simulink model "Car_Blinkers_2020b"  (R2020b)
settings: Solver=FixedStepDiscrete  StartTime=0.0  StopTime=10.0  FixedStep=1e-3  RelTol=1e-3
libraries: arduinolib x5, dspswit3 x3
settings Model: SILPILModeSetting=veronly  ExtModeTrigDuration=2  Creator=gaafa  LastModifiedBy=gaafa
settings SolverCC: AutoInsertRateTranBlk=on
settings OptimizationCC: UseDivisionForNetSlopeComputation=on  GainParamInheritBuiltInType=on  UseFloatMulNetSlope=on  PassReuseOutputArgsAs=Individual arguments  ZeroExternalMemoryAtStartup=off  ZeroInternalMemoryAtStartup=off  NoFixptDivByZeroProtection=on  EfficientFloat2IntCast=on  LifeSpan=1  MaxStackSize=64  OptimizeBlockOrder=speed  DifferentSizesBufferReuse=on  EfficientTunableParamExpr=on
settings DebuggingCC: ParameterTunabilityLossMsg=error  UnconnectedInputMsg=none  UnconnectedOutputMsg=none  UnconnectedLineMsg=none
settings HardwareCC: ProdBitPerInt=16  ProdBitPerPointer=16  ProdBitPerSizeT=16  ProdBitPerPtrDiffT=16  ProdLargestAtomicFloat=None  ProdWordSize=8  ProdHWDeviceType=Atmel->AVR
settings ModelReferenceCC: EnableRefExpFcnMdlSchedulingChecks=off
settings SFSimCC: MATLABDynamicMemAlloc=off
settings RTWCC: Description=Embedded Coder  SystemTargetFile=ert.tlc  HardwareBoard=Arduino Uno  TemplateMakefile=ert_default_tmf  Toolchain=Arduino AVR  BuildConfiguration=Faster Runs
settings CodeAppCC: ForceParamTrailComments=on  IgnoreCustomStorageClasses=off  OperatorAnnotations=on  SimulinkDataObjDesc=on  SFDataObjDesc=on  CustomSymbolStrGlobalVar=rt$N$M  CustomSymbolStrType=$N$M  CustomSymbolStrFcn=$N$M$F  CustomSymbolStrMacro=$N$M  InsertBlockDesc=on
settings ERTTargetCC: IncludeMdlTerminateFcn=off  CombineSignalStateStructs=on  SupportAbsoluteTime=off  SupportComplex=off  SupportContinuousTime=on  SupportNonInlinedSFcns=on  SupportVariableSizeSignals=on  ExtModeTransport=3  ExtModeStaticAlloc=on  ExtModeStaticAllocSize=250  ExtModeMexFile=ext_xcp  ExtModeIntrfLevel=Level2 - Open  ERTFilePackagingFormat=CompactWithDataFile

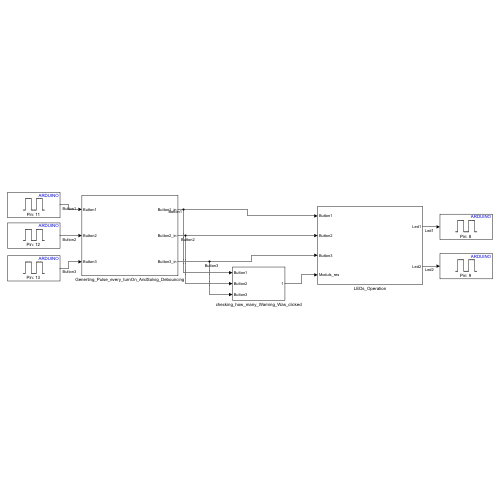
[thumbnail: Simulink's stored preview of the top-level diagram]
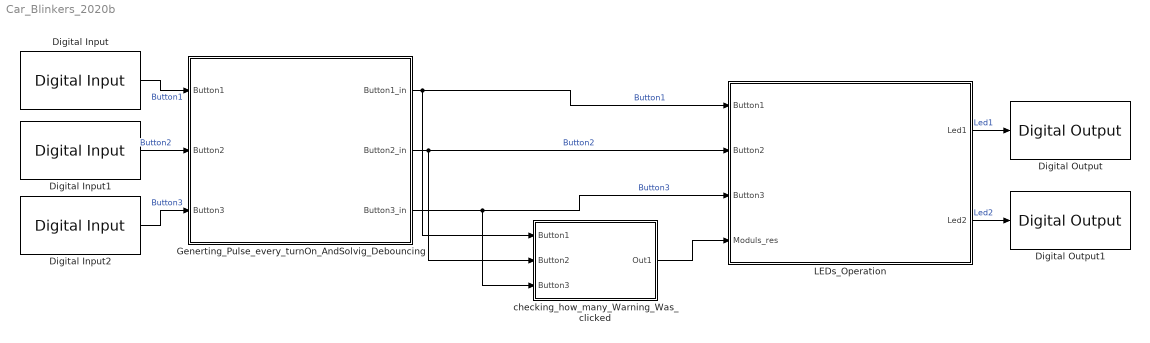
== system Car_Blinkers_2020b ==
  Digital Input : arduinolib/Digital Input  pinNumber=11  mode=Default  Direction=input  SampleTime=0.1  blockPlatform=arduino
  Digital Input1 : arduinolib/Digital Input  pinNumber=12  mode=Default  Direction=input  SampleTime=0.1  blockPlatform=arduino
  Digital Input2 : arduinolib/Digital Input  pinNumber=13  mode=Default  Direction=input  SampleTime=0.1  blockPlatform=arduino
  Digital Output : arduinolib/Digital Output  pinNumber=8  Direction=output  blockPlatform=arduino
  Digital Output1 : arduinolib/Digital Output  pinNumber=9  Direction=output  blockPlatform=arduino
  Generting_Pulse_every_turnOn_AndSolvig_Debouncing : Subsystem
  LEDs_Operation : Subsystem
  checking_how_many_Warning_Was_clicked : Subsystem
  wires:
  Digital Input/1 -> Generting_Pulse_every_turnOn_AndSolvig_Debouncing/1(Button1)  "Button1"
  Digital Input1/1 -> Generting_Pulse_every_turnOn_AndSolvig_Debouncing/2(Button2)  "Button2"
  LEDs_Operation/1(Led1) -> Digital Output/1  "Led1"
  Generting_Pulse_every_turnOn_AndSolvig_Debouncing/3(Button3_in) -> LEDs_Operation/3(Button3), checking_how_many_Warning_Was_clicked/3(Button3)  "Button3"
  Generting_Pulse_every_turnOn_AndSolvig_Debouncing/2(Button2_in) -> LEDs_Operation/2(Button2), checking_how_many_Warning_Was_clicked/2(Button2)  "Button2"
  Digital Input2/1 -> Generting_Pulse_every_turnOn_AndSolvig_Debouncing/3(Button3)  "Button3"
  Generting_Pulse_every_turnOn_AndSolvig_Debouncing/1(Button1_in) -> checking_how_many_Warning_Was_clicked/1(Button1), LEDs_Operation/1(Button1)  "Button1"
  checking_how_many_Warning_Was_clicked/1(Out1) -> LEDs_Operation/4(Moduls_res)
  LEDs_Operation/2(Led2) -> Digital Output1/1  "Led2"

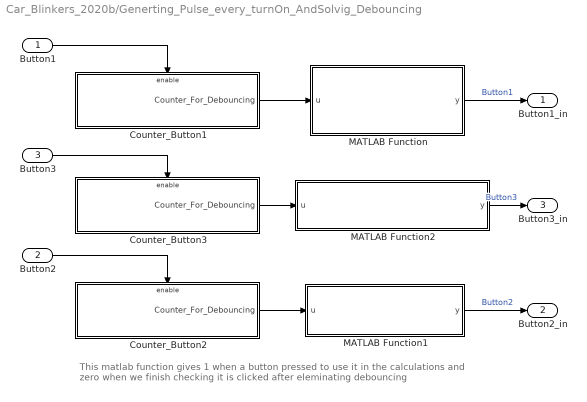
== system Car_Blinkers_2020b/Generting_Pulse_every_turnOn_AndSolvig_Debouncing ==
  note: This matlab function gives 1 when a button pressed to use it in the calculations
      | and zero when we finish checking it is clicked after eleminating debouncing
  Button1 : Inport
  Button2 : Inport  Port=2
  Button3 : Inport  Port=3
  Counter_Button1 : Subsystem  TreatAsAtomicUnit=on
  Counter_Button2 : Subsystem  TreatAsAtomicUnit=on
  Counter_Button3 : Subsystem  TreatAsAtomicUnit=on
  MATLAB Function : MATLAB Function  TreatAsAtomicUnit=on
  MATLAB Function1 : MATLAB Function  TreatAsAtomicUnit=on
  MATLAB Function2 : MATLAB Function  TreatAsAtomicUnit=on
  Button1_in : Outport
  Button2_in : Outport  Port=2
  Button3_in : Outport  Port=3
  wires:
  Counter_Button1/1(Counter_For_Debouncing) -> MATLAB Function/1(u)
  Button2/1 -> Counter_Button2/Enable
  Button3/1 -> Counter_Button3/Enable
  Button1/1 -> Counter_Button1/Enable
  Counter_Button3/1(Counter_For_Debouncing) -> MATLAB Function2/1(u)
  MATLAB Function2/1(y) -> Button3_in/1  "Button3"
  MATLAB Function/1(y) -> Button1_in/1  "Button1"
  Counter_Button2/1(Counter_For_Debouncing) -> MATLAB Function1/1(u)
  MATLAB Function1/1(y) -> Button2_in/1  "Button2"

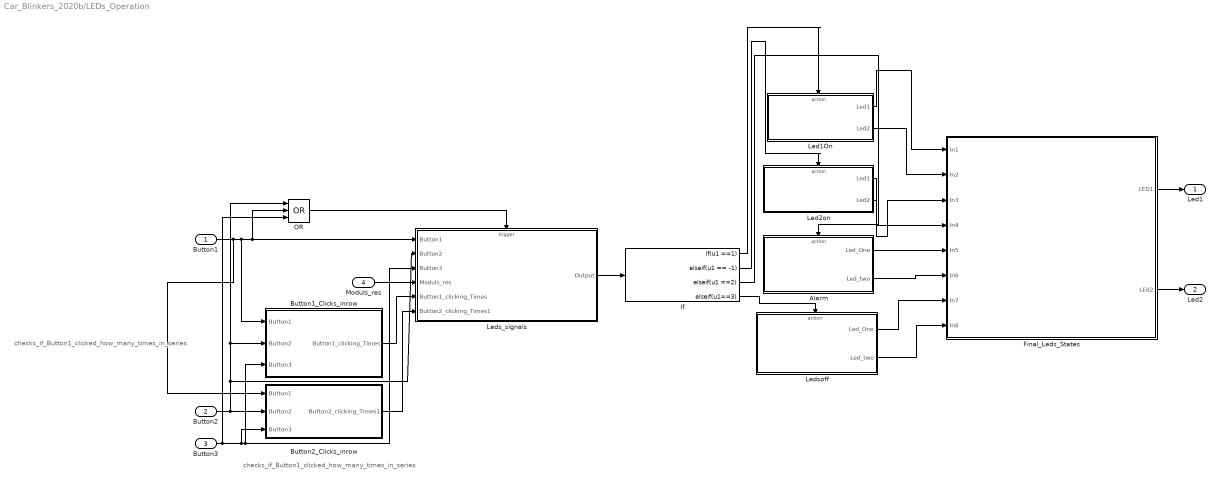
== system Car_Blinkers_2020b/LEDs_Operation ==
  note: checks_if_Button1_clicked_how_many_times_in_series
  note: checks_if_Button1_clicked_how_many_times_in_series
  Button1 : Inport
  Button2 : Inport  Port=2
  Button3 : Inport  Port=3
  Moduls_res : Inport  Port=4
  Alarm : Subsystem  TreatAsAtomicUnit=on
  Button1_Clicks_inrow : Subsystem
  Button2_Clicks_inrow : Subsystem
  Final_Leds_States : Subsystem
  If : If  IfExpression=u1 ==1  ElseIfExpressions=u1 == -1 , u1 ==2 , u1==3  ShowElse=off
  Led1On : Subsystem  TreatAsAtomicUnit=on
  Led2on : Subsystem  TreatAsAtomicUnit=on
  Leds_signals : Subsystem  TreatAsAtomicUnit=on
  Ledsoff : Subsystem  TreatAsAtomicUnit=on
  OR : Logic  Operator=OR  Inputs=3  IconShape=distinctive  AllPortsSameDT=off  OutDataTypeStr=boolean
  Led1 : Outport
  Led2 : Outport  Port=2
  wires:
  If/4 -> Ledsoff/Action
  Button1/1 -> OR/2, Leds_signals/1(Button1), Button1_Clicks_inrow/1(Button1), Button2_Clicks_inrow/1(Button1)
  Moduls_res/1 -> Leds_signals/4(Moduls_res)
  Button2/1 -> Button1_Clicks_inrow/2(Button2), OR/1, Leds_signals/2(Button2), Button2_Clicks_inrow/2(Button2)
  Leds_signals/1(Output) -> If/1
  Button2_Clicks_inrow/1(Button2_clicking_Times1) -> Leds_signals/6(Button2_clicking_Times1)
  Button3/1 -> Button1_Clicks_inrow/3(Button3), Leds_signals/3(Button3), Button2_Clicks_inrow/3(Button3), OR/3
  OR/1 -> Leds_signals/Trigger
  Final_Leds_States/1(LED1) -> Led1/1
  Led2on/2(Led2) -> Final_Leds_States/4(In4)
  Button1_Clicks_inrow/1(Button1_clicking_Times) -> Leds_signals/5(Button1_clicking_Times)
  If/1 -> Led1On/Action
  Alarm/2(Led_two) -> Final_Leds_States/6(In6)
  If/2 -> Led2on/Action
  If/3 -> Alarm/Action
  Ledsoff/2(Led_two) -> Final_Leds_States/8(In8)
  Led1On/1(Led1) -> Final_Leds_States/1(In1)
  Led1On/2(Led2) -> Final_Leds_States/2(In2)
  Led2on/1(Led1) -> Final_Leds_States/3(In3)
  Alarm/1(Led_One) -> Final_Leds_States/5(In5)
  Ledsoff/1(Led_One) -> Final_Leds_States/7(In7)
  Final_Leds_States/2(LEd2) -> Led2/1

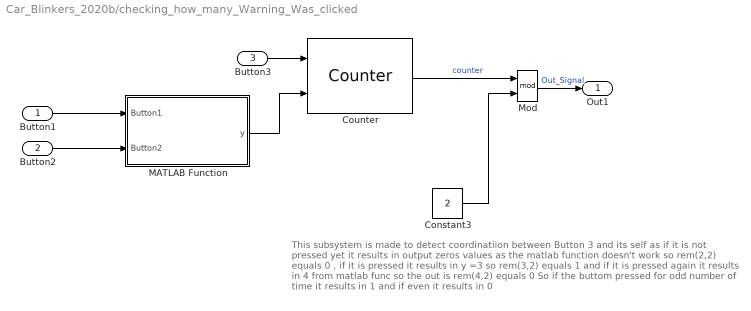
== system Car_Blinkers_2020b/checking_how_many_Warning_Was_clicked ==
  note: This subsystem is made to detect coordinatiion between Button 3 and its self as if it is not pressed yet it results in output zeros values as the matlab function doesn't work
      | so rem(2,2) equals 0 , if it is pressed it results in y =3 so rem(3,2) equals 1 and if it is pressed again it results in 4 from matlab func so the out is rem(4,2) equals 0
      | So if the buttom pressed for odd number of time it results in 1 and if even it results in 0
  Button1 : Inport
  Button2 : Inport  Port=2
  Button3 : Inport  Port=3
  Constant3 : Constant  Value=2
  Counter : dspswit3/Counter  Direction=Up  CountEvent=Rising edge  CounterSize=User defined  MaxCount=255  InitialCount=0  Output=Count  HitValue=32  ResetInput=on  SamplesPerFrame=1  Ts=1  CntDtype=double  HitDtype=Logical
  MATLAB Function : MATLAB Function  TreatAsAtomicUnit=on
  Mod : Math  Operator=mod  SaturateOnIntegerOverflow=on
  Out1 : Outport
  wires:
  Constant3/1 -> Mod/2
  Counter/1 -> Mod/1  "counter"
  Button3/1 -> Counter/1
  Mod/1 -> Out1/1  "Out_Signal"
  MATLAB Function/1(y) -> Counter/2
  Button2/1 -> MATLAB Function/2(Button2)
  Button1/1 -> MATLAB Function/1(Button1)

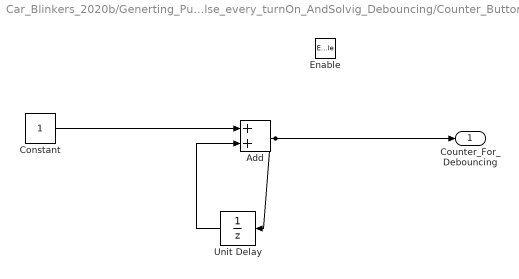
== system Car_Blinkers_2020b/Generting_Pulse_every_turnOn_AndSolvig_Debouncing/Counter_Button1 ==
  Enable : EnablePort  StatesWhenEnabling=reset
  Add : Sum
  Constant : Constant
  Unit Delay : UnitDelay  SampleTime=1e-3  HasFrameUpgradeWarning=on
  Counter_For_Debouncing : Outport
  wires:
  Constant/1 -> Add/1
  Unit Delay/1 -> Add/2
  Add/1 -> Unit Delay/1, Counter_For_Debouncing/1

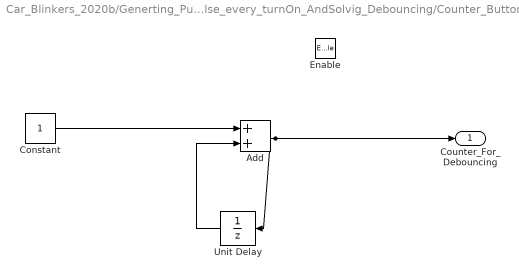
== system Car_Blinkers_2020b/Generting_Pulse_every_turnOn_AndSolvig_Debouncing/Counter_Button2 ==
  Enable : EnablePort  StatesWhenEnabling=reset
  Add : Sum
  Constant : Constant
  Unit Delay : UnitDelay  SampleTime=1e-3  HasFrameUpgradeWarning=on
  Counter_For_Debouncing : Outport
  wires:
  Add/1 -> Counter_For_Debouncing/1, Unit Delay/1
  Unit Delay/1 -> Add/2
  Constant/1 -> Add/1

== system Car_Blinkers_2020b/Generting_Pulse_every_turnOn_AndSolvig_Debouncing/Counter_Button3 ==
  Enable : EnablePort  StatesWhenEnabling=reset
  Add : Sum
  Constant : Constant
  Unit Delay : UnitDelay  SampleTime=1e-3  HasFrameUpgradeWarning=on
  Counter_For_Debouncing : Outport
  wires:
  Constant/1 -> Add/1
  Unit Delay/1 -> Add/2
  Add/1 -> Unit Delay/1, Counter_For_Debouncing/1

== system Car_Blinkers_2020b/LEDs_Operation/Alarm ==
  Action Port : ActionPort  ActionPortLabel=elseif( u1 ==2 )
  Constant : Constant
  Constant1 : Constant
  Led_One : Outport
  Led_two : Outport  Port=2
  wires:
  Constant/1 -> Led_One/1
  Constant1/1 -> Led_two/1

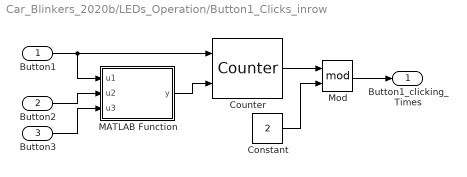
== system Car_Blinkers_2020b/LEDs_Operation/Button1_Clicks_inrow ==
  Button1 : Inport
  Button2 : Inport  Port=2
  Button3 : Inport  Port=3
  Constant : Constant  Value=2
  Counter : dspswit3/Counter  Direction=Up  CountEvent=Rising edge  CounterSize=User defined  MaxCount=255  InitialCount=0  Output=Count  HitValue=32  ResetInput=on  SamplesPerFrame=1  Ts=1  CntDtype=double  HitDtype=Logical
  MATLAB Function : MATLAB Function  TreatAsAtomicUnit=on
  Mod : Math  Operator=mod  SaturateOnIntegerOverflow=on
  Button1_clicking_Times : Outport
  wires:
  Button2/1 -> MATLAB Function/2(u2)
  Button1/1 -> Counter/1, MATLAB Function/1(u1)
  MATLAB Function/1(y) -> Counter/2
  Counter/1 -> Mod/1
  Mod/1 -> Button1_clicking_Times/1
  Constant/1 -> Mod/2
  Button3/1 -> MATLAB Function/3(u3)

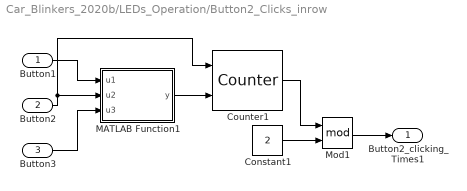
== system Car_Blinkers_2020b/LEDs_Operation/Button2_Clicks_inrow ==
  Button1 : Inport
  Button2 : Inport  Port=2
  Button3 : Inport  Port=3
  Constant1 : Constant  Value=2
  Counter1 : dspswit3/Counter  Direction=Up  CountEvent=Rising edge  CounterSize=User defined  MaxCount=255  InitialCount=0  Output=Count  HitValue=32  ResetInput=on  SamplesPerFrame=1  Ts=1  CntDtype=double  HitDtype=Logical
  MATLAB Function1 : MATLAB Function  TreatAsAtomicUnit=on
  Mod1 : Math  Operator=mod  SaturateOnIntegerOverflow=on
  Button2_clicking_Times1 : Outport
  wires:
  Button2/1 -> Counter1/1, MATLAB Function1/2(u2)
  Button1/1 -> MATLAB Function1/1(u1)
  MATLAB Function1/1(y) -> Counter1/2
  Mod1/1 -> Button2_clicking_Times1/1
  Constant1/1 -> Mod1/2
  Counter1/1 -> Mod1/1
  Button3/1 -> MATLAB Function1/3(u3)

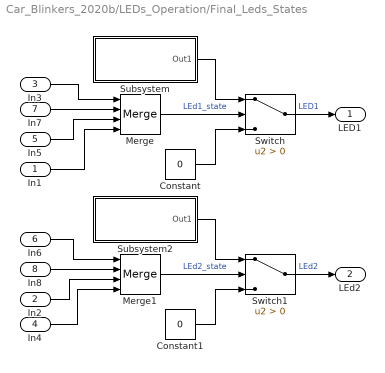
== system Car_Blinkers_2020b/LEDs_Operation/Final_Leds_States ==
  In1 : Inport
  In2 : Inport  Port=2
  In3 : Inport  Port=3
  In4 : Inport  Port=4
  In5 : Inport  Port=5
  In6 : Inport  Port=6
  In7 : Inport  Port=7
  In8 : Inport  Port=8
  Constant : Constant  Value=0
  Constant1 : Constant  Value=0
  Merge : Merge  Inputs=4
  Merge1 : Merge  Inputs=4
  Subsystem : Subsystem
  Subsystem2 : Subsystem
  Switch : Switch  Criteria=u2 > Threshold
  Switch1 : Switch  Criteria=u2 > Threshold
  LED1 : Outport
  LEd2 : Outport  Port=2
  wires:
  In8/1 -> Merge1/2
  In3/1 -> Merge/1
  In7/1 -> Merge/2
  In4/1 -> Merge1/4
  Merge1/1 -> Switch1/2  "LEd2_state"
  In2/1 -> Merge1/3
  In1/1 -> Merge/4
  In5/1 -> Merge/3
  Switch/1 -> LED1/1  "LED1"
  In6/1 -> Merge1/1
  Subsystem/1(Out1) -> Switch/1
  Merge/1 -> Switch/2  "LEd1_state"
  Constant/1 -> Switch/3
  Subsystem2/1(Out1) -> Switch1/1
  Constant1/1 -> Switch1/3
  Switch1/1 -> LEd2/1  "LEd2"

== system Car_Blinkers_2020b/LEDs_Operation/Led1On ==
  Action Port : ActionPort  ActionPortLabel=if(u1 ==1)
  Constant : Constant
  Constant1 : Constant  Value=0
  Led1 : Outport
  Led2 : Outport  Port=2
  wires:
  Constant/1 -> Led1/1
  Constant1/1 -> Led2/1

== system Car_Blinkers_2020b/LEDs_Operation/Led2on ==
  Action Port : ActionPort  ActionPortLabel=elseif(u1 == -1 )
  Constant : Constant  Value=0
  Constant1 : Constant
  Led1 : Outport
  Led2 : Outport  Port=2
  wires:
  Constant/1 -> Led1/1
  Constant1/1 -> Led2/1

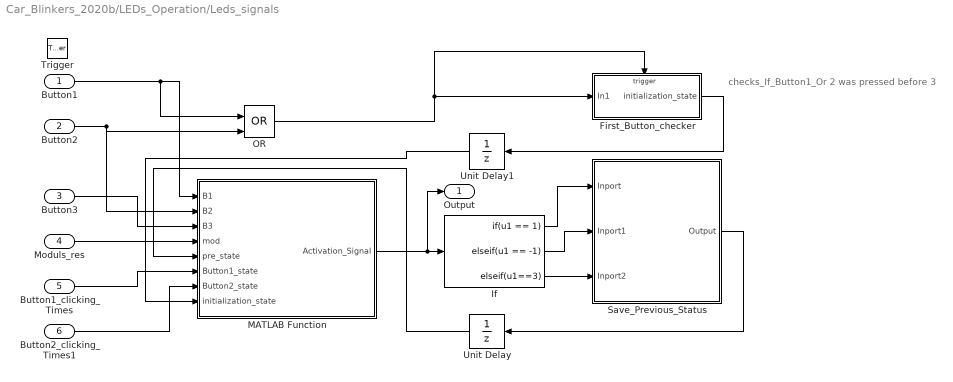
== system Car_Blinkers_2020b/LEDs_Operation/Leds_signals ==
  note: checks_If_Button1_Or 2 was pressed before 3
  Button1 : Inport
  Button2 : Inport  Port=2
  Button3 : Inport  Port=3
  Moduls_res : Inport  Port=4
  Button1_clicking_Times : Inport  Port=5
  Button2_clicking_Times1 : Inport  Port=6
  Trigger : TriggerPort  VariantControl=(inherit)  PortDimensions=1
  First_Button_checker : Subsystem  TreatAsAtomicUnit=on
  If : If  IfExpression=u1 == 1  ElseIfExpressions=u1 == -1 , u1==3  ShowElse=off
  MATLAB Function : MATLAB Function  TreatAsAtomicUnit=on
  OR : Logic  Operator=OR  IconShape=distinctive  AllPortsSameDT=off  OutDataTypeStr=boolean
  Save_Previous_Status : Subsystem
  Unit Delay : UnitDelay  SampleTime=-1  HasFrameUpgradeWarning=on
  Unit Delay1 : UnitDelay  SampleTime=-1  HasFrameUpgradeWarning=on
  Output : Outport
  wires:
  Button1_clicking_Times/1 -> MATLAB Function/6(Button1_state)
  Button3/1 -> MATLAB Function/3(B3)
  Button1/1 -> OR/1, MATLAB Function/1(B1)
  MATLAB Function/1(Activation_Signal) -> Output/1, If/1
  Button2/1 -> OR/2, MATLAB Function/2(B2)
  Unit Delay/1 -> MATLAB Function/5(pre_state)
  OR/1 -> First_Button_checker/1(In1), First_Button_checker/Trigger
  Moduls_res/1 -> MATLAB Function/4(mod)
  Button2_clicking_Times1/1 -> MATLAB Function/7(Button2_state)
  Unit Delay1/1 -> MATLAB Function/8(initialization_state)
  If/1 -> Save_Previous_Status/1(Inport)
  If/2 -> Save_Previous_Status/2(Inport1)
  If/3 -> Save_Previous_Status/3(Inport2)
  First_Button_checker/1(initialization_state) -> Unit Delay1/1
  Save_Previous_Status/1(Output) -> Unit Delay/1

== system Car_Blinkers_2020b/LEDs_Operation/Ledsoff ==
  Action Port : ActionPort  ActionPortLabel=elseif( u1==3)
  Constant : Constant  Value=0
  Constant1 : Constant  Value=0
  Led_One : Outport
  Led_two : Outport  Port=2
  wires:
  Constant/1 -> Led_One/1
  Constant1/1 -> Led_two/1

== system Car_Blinkers_2020b/LEDs_Operation/Final_Leds_States/Subsystem ==
  AND : Logic  IconShape=distinctive  AllPortsSameDT=off  OutDataTypeStr=boolean
  Constant : Constant
  NOT : Logic  Operator=NOT  IconShape=distinctive  AllPortsSameDT=off  OutDataTypeStr=boolean
  Unit Delay : UnitDelay  InitialCondition=1  SampleTime=0.4  HasFrameUpgradeWarning=on
  Out1 : Outport
  wires:
  Constant/1 -> AND/1
  AND/1 -> Unit Delay/1, Out1/1
  Unit Delay/1 -> NOT/1
  NOT/1 -> AND/2

== system Car_Blinkers_2020b/LEDs_Operation/Final_Leds_States/Subsystem2 ==
  AND : Logic  IconShape=distinctive  AllPortsSameDT=off  OutDataTypeStr=boolean
  Constant : Constant
  NOT : Logic  Operator=NOT  IconShape=distinctive  AllPortsSameDT=off  OutDataTypeStr=boolean
  Unit Delay : UnitDelay  InitialCondition=1  SampleTime=0.4  HasFrameUpgradeWarning=on
  Out1 : Outport
  wires:
  NOT/1 -> AND/2
  Unit Delay/1 -> NOT/1
  AND/1 -> Out1/1, Unit Delay/1
  Constant/1 -> AND/1

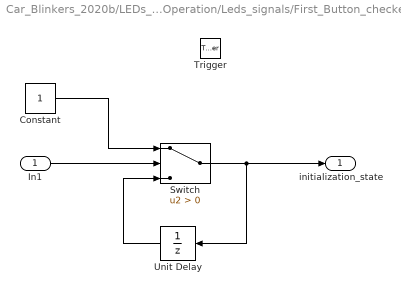
== system Car_Blinkers_2020b/LEDs_Operation/Leds_signals/First_Button_checker ==
  In1 : Inport
  Trigger : TriggerPort  VariantControl=(inherit)
  Constant : Constant
  Switch : Switch  Criteria=u2 > Threshold
  Unit Delay : UnitDelay  SampleTime=-1  HasFrameUpgradeWarning=on
  initialization_state : Outport
  wires:
  In1/1 -> Switch/2
  Constant/1 -> Switch/1
  Switch/1 -> Unit Delay/1, initialization_state/1
  Unit Delay/1 -> Switch/3

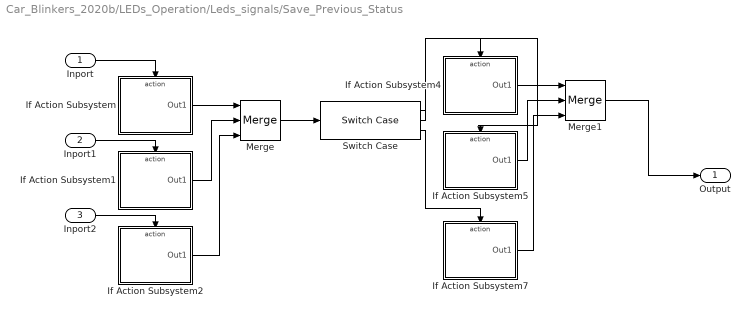
== system Car_Blinkers_2020b/LEDs_Operation/Leds_signals/Save_Previous_Status ==
  Inport : Inport
  Inport1 : Inport  Port=2
  Inport2 : Inport  Port=3
  If Action Subsystem : Subsystem  TreatAsAtomicUnit=on
  If Action Subsystem1 : Subsystem  TreatAsAtomicUnit=on
  If Action Subsystem2 : Subsystem  TreatAsAtomicUnit=on
  If Action Subsystem4 : Subsystem  TreatAsAtomicUnit=on
  If Action Subsystem5 : Subsystem  TreatAsAtomicUnit=on
  If Action Subsystem7 : Subsystem  TreatAsAtomicUnit=on
  Merge : Merge  Inputs=3
  Merge1 : Merge  Inputs=3
  Switch Case : SwitchCase  CaseConditions="{1  ;-1  ;3}"  ShowDefaultCase=off
  Output : Outport
  wires:
  Inport/1 -> If Action Subsystem/Action
  If Action Subsystem1/1(Out1) -> Merge/2
  If Action Subsystem5/1(Out1) -> Merge1/2
  Inport1/1 -> If Action Subsystem1/Action
  Merge/1 -> Switch Case/1
  Inport2/1 -> If Action Subsystem2/Action
  Merge1/1 -> Output/1
  If Action Subsystem/1(Out1) -> Merge/1
  If Action Subsystem2/1(Out1) -> Merge/3
  Switch Case/1 -> If Action Subsystem4/Action
  Switch Case/2 -> If Action Subsystem5/Action
  Switch Case/3 -> If Action Subsystem7/Action
  If Action Subsystem4/1(Out1) -> Merge1/1
  If Action Subsystem7/1(Out1) -> Merge1/3

== system Car_Blinkers_2020b/LEDs_Operation/Leds_signals/Save_Previous_Status/If Action Subsystem ==
  Action Port : ActionPort  ActionPortLabel=if(u1 == 1)
  Constant : Constant
  Out1 : Outport
  wires:
  Constant/1 -> Out1/1

== system Car_Blinkers_2020b/LEDs_Operation/Leds_signals/Save_Previous_Status/If Action Subsystem1 ==
  Action Port : ActionPort  ActionPortLabel=elseif(u1 == -1 )
  Constant : Constant  Value=-1
  Out1 : Outport
  wires:
  Constant/1 -> Out1/1

== system Car_Blinkers_2020b/LEDs_Operation/Leds_signals/Save_Previous_Status/If Action Subsystem2 ==
  Action Port : ActionPort  ActionPortLabel=elseif( u1==3 )
  Constant : Constant  Value=3
  Out1 : Outport
  wires:
  Constant/1 -> Out1/1

== system Car_Blinkers_2020b/LEDs_Operation/Leds_signals/Save_Previous_Status/If Action Subsystem4 ==
  Action Port : ActionPort  ActionPortLabel=case [ 1 ]:
  Constant : Constant
  Out1 : Outport
  wires:
  Constant/1 -> Out1/1

== system Car_Blinkers_2020b/LEDs_Operation/Leds_signals/Save_Previous_Status/If Action Subsystem5 ==
  Action Port : ActionPort  ActionPortLabel=case [ -1 ]:
  Constant : Constant  Value=-1
  Out1 : Outport
  wires:
  Constant/1 -> Out1/1

== system Car_Blinkers_2020b/LEDs_Operation/Leds_signals/Save_Previous_Status/If Action Subsystem7 ==
  Action Port : ActionPort  ActionPortLabel=case [ 3 ]:
  Constant : Constant  Value=3
  Out1 : Outport
  wires:
  Constant/1 -> Out1/1

== matlab function Car_Blinkers_2020b/Generting_Pulse_every_turnOn_AndSolvig_Debouncing/MATLAB Function2 ==
  data: u input; y output
function y = Checking_Button_pushing(u)
y=0;
if (u ==10)
    y=1;
end

== matlab function Car_Blinkers_2020b/checking_how_many_Warning_Was_clicked/MATLAB Function ==
  data: Button1 input; y output; Button2 input
function y = fcn(Button1 , Button2)
y=0
if (Button1==1 | Button2 ==1)
    y=1;
end

== matlab function Car_Blinkers_2020b/Generting_Pulse_every_turnOn_AndSolvig_Debouncing/MATLAB Function ==
  data: u input; y output
function y = Checking_Button_pushing(u)
y=0;
if (u ==10)
    y=1;
end

== matlab function Car_Blinkers_2020b/Generting_Pulse_every_turnOn_AndSolvig_Debouncing/MATLAB Function1 ==
  data: u input; y output
function y = Checking_Button_pushing(u)
y=0;
if (u ==10)
    y=1;
end

== matlab function Car_Blinkers_2020b/LEDs_Operation/Leds_signals/MATLAB Function ==
  data: B1 input; Activation_Signal output; B2 input; B3 input; mod input; pre_state input; Button1_state input; Button2_state input; initialization_state input
function Activation_Signal = fcn(B1 , B2 , B3 ,mod,pre_state , Button1_state , Button2_state , initialization_state)

Activation_Signal = 0;

if (B1 == 1 && B2 ==0 && B3 == 0 && Button1_state ~=0)%Button1 is on so blink Led 1
    Activation_Signal = 1;
elseif ( (B1 == 1 && B2 ==0 && B3 == 0 && Button1_state ==0) || (B1 == 0 && B2 ==1 && B3 == 0 && Button2_state ==0) )%This line is made to handle if I pressed on button1 or 2 again to turn led off
    Activation_Signal = 3;
elseif( B1 == 0 && B2 ==1 && B3 == 0 && Button2_state ~=0 )%Button2 is on so blink Led 2
    Activation_Signal = -1;
elseif (B1 == 0 && B2 ==0 && mod ==1) %Button3 is on so blink an alarm
    Activation_Signal = 2;
elseif (B1 == 0 && B2 ==0 && mod ==0) %Button3 is on again so stop an alarm
    Activation_Signal = pre_state;
end

if (initialization_state == 0 && mod == 0 && pre_state ==0 && B1 == 0 && B2 ==0)% This line is made to handle that case if Alarm was fired at first and need to be back to the state before, This make u return to leds off

    Activation_Signal = 3;
end

if (pre_state == -1 && Button2_state ~=0) %These 2 lines are witten to handle if I return to previous state in which B1 or B2 were on and I needed to turn them off by clicking buttons
    Activation_Signal =3;
end
if (pre_state == 1 && Button1_state ~=0)
    Activation_Signal =3;
end

== matlab function Car_Blinkers_2020b/LEDs_Operation/Button2_Clicks_inrow/MATLAB Function1 ==
  data: u1 input; y output; u2 input; u3 input
function y = fcn(u1 , u2 , u3 )
y = 0;
if (u1==0 & u2==1 & u3 ==0)
    y=0;
elseif (u1==1 & u2==0 | u3 ==1)
    y=1;
end

== matlab function Car_Blinkers_2020b/LEDs_Operation/Button1_Clicks_inrow/MATLAB Function ==
  data: u1 input; y output; u2 input; u3 input
function y = fcn(u1 , u2 , u3)
y = 0;
if (u1==1 & u2==0 & u3 ==0)
    y=0;
elseif (u1==0 & (u2==1 | u3 ==1 ))
    y=1;
end
